simulink model "Animate"  (R2014a)
settings: Solver=FixedStepDiscrete  StartTime=0.0  StopTime=tend  FixedStep=ts  RelTol=1e-3
InitFcn:
  | InitParams
values from neighbouring files (symbols this model uses):
  tslow = 1.0/50.0    (= 0.02)    [InitParams.m]    (also in InitParams4.m)
settings Model: Creator=etreadwa  LastModifiedBy=etreadwa
settings DataIOCC: LimitDataPoints=off  SaveOutput=off  SignalLogging=off  DSMLogging=off  SaveTime=off
settings DebuggingCC: ArrayBoundsChecking=warning  MergeDetectMultiDrivingBlocksExec=error  ParameterUnderflowMsg=warning  UnnecessaryDatatypeConvMsg=warning  VectorMatrixConversionMsg=warning  SFcnCompatibilityMsg=warning
settings HardwareCC: ProdHWDeviceType=Generic->Unspecified (assume 32-bit Generic)

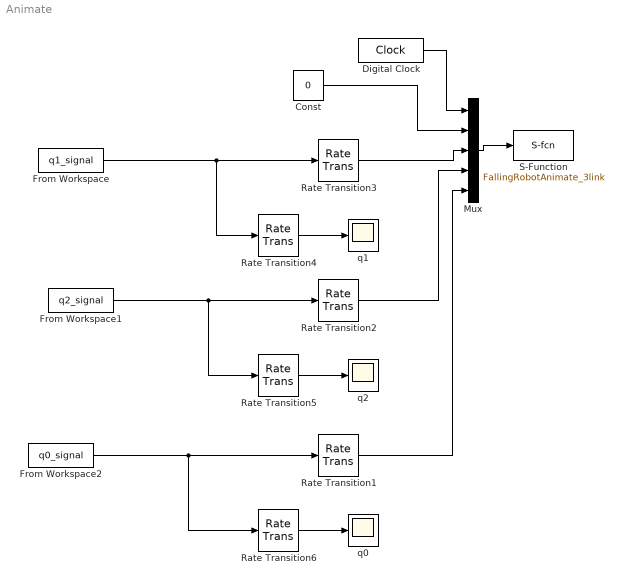
== system Animate ==
  Const : Constant  Value=0
  Digital Clock : DigitalClock  SampleTime=tslow
  From Workspace : FromWorkspace  VariableName=q1_signal  SampleTime=0
  From Workspace1 : FromWorkspace  VariableName=q2_signal  SampleTime=0
  From Workspace2 : FromWorkspace  VariableName=q0_signal  SampleTime=0
  Mux : Mux  Inputs=5
  Rate Transition{1..6} (6 alike) : RateTransition
  S-Function : S-Function  FunctionName=FallingRobotAnimate_3link  Parameters=tslow  EnableBusSupport=off
  q0 : Scope
      settings: YMin=-700  YMax=900  SaveName=q0  SampleInput=on  SampleTime=tsdata
  q1 : Scope
      settings: YMin=-700  YMax=900  SaveName=q1  SampleInput=on  SampleTime=tsdata
  q2 : Scope
      settings: YMin=-700  YMax=900  SaveName=q2  SampleInput=on  SampleTime=tsdata
  wires:
  Mux/1 -> S-Function/1
  Digital Clock/1 -> Mux/1
  Const/1 -> Mux/2
  Rate Transition4/1 -> q1/1
  Rate Transition5/1 -> q2/1
  Rate Transition3/1 -> Mux/3
  Rate Transition2/1 -> Mux/4
  Rate Transition6/1 -> q0/1
  Rate Transition1/1 -> Mux/5
  From Workspace/1 -> Rate Transition4/1, Rate Transition3/1
  From Workspace1/1 -> Rate Transition5/1, Rate Transition2/1
  From Workspace2/1 -> Rate Transition6/1, Rate Transition1/1
